simulink model "mcb_pmsm_foc_hall_f28379d"  (R2023b)
settings: Solver=FixedStepDiscrete  StartTime=0.0  StopTime=8  RelTol=1e-3  EnableMultiTasking=on
InitFcn:
  | mcb_pmsm_foc_hall_f28379d_data;
model workspace (MAT data in the model file):
  encoderResolution = 2000
  hallOffset = '0.5'
  indexOffset = 850
  polePairs = '4'
values from neighbouring files (symbols this model uses):
  dataType = 'single'    [mcb_pmsm_foc_hall_f28069m_data.m]    (also in mcb_pmsm_foc_hall_f28379d_data.m)
  inverter = mcb_SetInverterParameters('DRV8312-C2-KIT')    [mcb_pmsm_foc_hall_f28069m_data.m]    (also in mcb_pmsm_foc_hall_f28379d_data.m = mcb_updateInverterParameters(pmsm,inverter,target))
  PI_params = mcb_SetControllerParameters(pmsm,inverter,PU_System,T_pwm,Ts,Ts_speed)    [mcb_pmsm_foc_hall_f28069m_data.m]    (also in mcb_pmsm_foc_hall_f28379d_data.m)
  pmsm = mcb_SetPMSMMotorParameters('BLY171D')    [mcb_pmsm_foc_hall_f28069m_data.m]    (also in mcb_pmsm_foc_hall_f28379d_data.m = mcb_SetPMSMMotorParameters('custom'))
  PU_System = mcb_SetPUSystem(pmsm,inverter)    [mcb_pmsm_foc_hall_f28069m_data.m]    (also in mcb_pmsm_foc_hall_f28379d_data.m)
  target = mcb_SetProcessorDetails('F28069M',PWM_frequency)    [mcb_pmsm_foc_hall_f28069m_data.m]    (also in mcb_pmsm_foc_hall_f28379d_data.m = mcb_SetProcessorDetails('F28379D',PWM_frequency))
  Ts = T_pwm    (= 5e-05)    [mcb_pmsm_foc_hall_f28069m_data.m]    (also in mcb_pmsm_foc_hall_f28379d_data.m)
  Ts_motor = T_pwm/2    (= 2.5e-05)    [mcb_pmsm_foc_hall_f28069m_data.m]    (also in mcb_pmsm_foc_hall_f28379d_data.m)
  Ts_simulink = T_pwm/2    (= 2.5e-05)    [mcb_pmsm_foc_hall_f28069m_data.m]    (also in mcb_pmsm_foc_hall_f28379d_data.m)
  Ts_speed = 10*Ts    (= 0.0005)    [mcb_pmsm_foc_hall_f28069m_data.m]    (also in mcb_pmsm_foc_hall_f28379d_data.m)
undefined symbols (not defined in the file or in its folder): DiscIntNeverNeededParam, Down, GPTRIP1SEL, GPTRIP2SEL, Ts_sensor, TZ1, TZ2, Up
libraries: simulink x37, mcbpositiondecoderlib x12, mcbcontrolslib x11, idelinklib_common x8, c280xlib x8, c2802xlib x7, svdschedulerlib x5, slpidlib x4, c2837xDlib x3, svdutilitieslib x1, mcbplantlib x1, autolibpmsmexterior x1
(part 2 of 4)

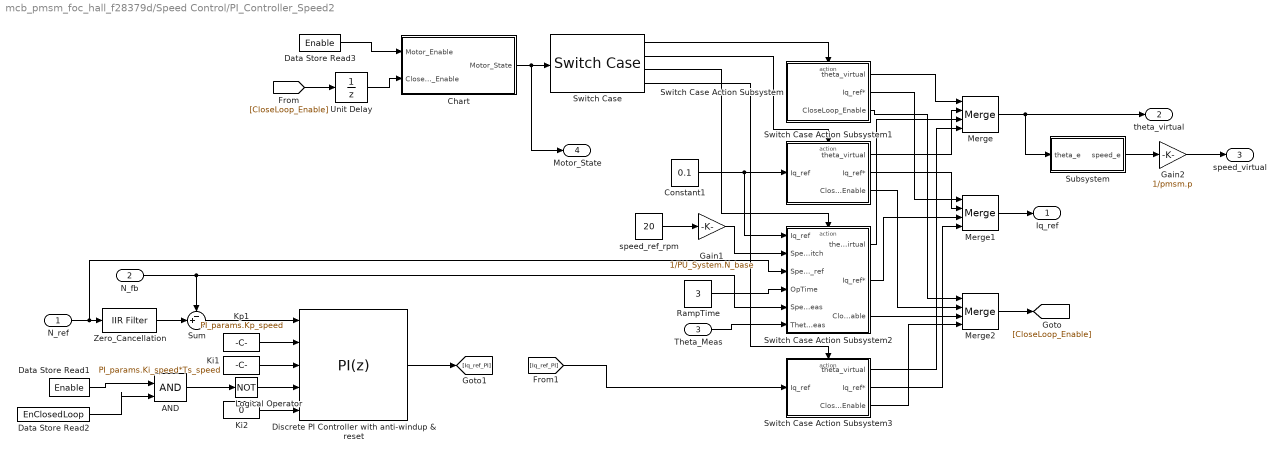
== system mcb_pmsm_foc_hall_f28379d/Speed Control/PI_Controller_Speed2 ==
  N_ref : Inport
  N_fb : Inport  Port=2
  Theta_Meas : Inport  Port=3
  AND : Logic  IconShape=distinctive  AllPortsSameDT=off  OutDataTypeStr=boolean
  Chart : Stateflow chart  TreatAsAtomicUnit=on
  Constant1 : Constant  Value=0.1  OutDataTypeStr=single
  Data Store Read2 : DataStoreRead  DataStoreName=EnClosedLoop  IndexOptions=Index vector (dialog)  Indices=1  OutputSizes=1
  Data Store Read1 : DataStoreRead  DataStoreName=Enable  IndexOptions=Index vector (dialog)  Indices=1  OutputSizes=1
  Data Store Read3 : DataStoreRead  DataStoreName=Enable  IndexOptions=Index vector (dialog)  Indices=1  OutputSizes=1
  Discrete PI Controller with anti-windup & reset : slpidlib/PID Controller  Controller=PI  Form=Parallel  TimeDomain=Discrete-time  UseExternalTs=off  SampleTime=-1  IntegratorMethod=Forward Euler  FilterMethod=Forward Euler  ControllerParametersSource=external  P=1  I=1  UseKiTs=on  D=0  N=100  UseFilter=on  TunerSelectOption=Transfer Function Based (PID Tuner App)  InitialConditionSource=external  InitialConditionForIntegrator=0  InitialConditionForFilter=0  DifferentiatorICPrevScaledInput=0  ExternalReset=level  TrackingMode=off  Kt=1  LimitOutput=on  SatLimitsSource=internal  UpperSaturationLimit=1  LowerSaturationLimit=-1  LinearizeAsGain=on  AntiWindupMode=clamping  Kb=1  LimitIntegrator=off  UpperIntegratorSaturationLimit=inf  LowerIntegratorSaturationLimit=-inf  RndMeth=Simplest  POutMin=[]  POutMax=[]  IOutMin=[]  IOutMax=[]  DOutMin=[]  DOutMax=[]  NOutMin=[]  NOutMax=[]  SumOutMin=[]  SumOutMax=[]  SaturationOutDataTypeStr=Inherit: Inherit via back propagation  SaturationOutMin=[]  SaturationOutMax=[]  PParamMin=[]  PParamMax=[]  IParamMin=[]  IParamMax=[]  DParamMin=[]  DParamMax=[]  NParamMin=[]  NParamMax=[]  KbParamMin=[]  KbParamMax=[]  KtParamMin=[]  KtParamMax=[]  KbOutMin=[]  KbOutMax=[]  KtOutMin=[]  KtOutMax=[]  IntegratorOutMin=[]  IntegratorOutMax=[]  FilterOutMin=[]  FilterOutMax=[]  SumI1OutMin=[]  SumI1OutMax=[]  SumI2OutMin=[]  SumI2OutMax=[]  SumI3OutMin=[]  SumI3OutMax=[]  SumI4OutMin=[]  SumI4OutMax=[]  SumDOutMin=[]  SumDOutMax=[]  DifferentiatorOutMin=[]  DifferentiatorOutMax=[]  FilterDiffOutCoefMin=[]  FilterDiffOutCoefMax=[]  ReciprocalOutMin=[]  ReciprocalOutMax=[]  SumDenOutMin=[]  SumDenOutMax=[]  SumNumOutMin=[]  SumNumOutMax=[]  DivideOutMin=[]  DivideOutMax=[]  UdiffTsProdOutMin=[]  UdiffTsProdOutMax=[]  NTsProdOutMin=[]  NTsProdOutMax=[]  UintegralTsProdOutMin=[]  UintegralTsProdOutMax=[]  UngainTsProdOutMin=[]  UngainTsProdOutMax=[]  ClampingZeroOutDataTypeStr=Inherit: Inherit via back propagation  ClampingZeroOutMin=[]  ClampingZeroOutMax=[]  FilterDenConstantOutDataTypeStr=Inherit: Inherit via back propagation  FilterDenConstantOutMin=[]  FilterDenConstantOutMax=[]  PCopyOutDataTypeStr=Inherit: Inherit via back propagation  PCopyOutMin=[]  PCopyOutMax=[]  NCopyOutDataTypeStr=Inherit: Inherit via back propagation  NCopyOutMin=[]  NCopyOutMax=[]  IntegratorContinuousStateAttributes=''  IntegratorStateMustResolveToSignalObject=off  IntegratorRTWStateStorageClass=Auto  FilterContinuousStateAttributes=''  FilterStateMustResolveToSignalObject=off  FilterRTWStateStorageClass=Auto  ParallelPVariant=ExternalParameters  IdealPVariant=Disabled  IVariant=ExternalParameters  DVariant=Disabled  IntegratorVariant=Discrete  SatVariant=Enabled  AWVariant=DiscClampingParallel  PCopyVariant=Disabled  TRVariant=Disabled  FdbkBlocksVariant=Forward  IdealPFdbkVariant=Disabled  SatFdbkVariant=Disabled  DerivativeFilterVariant=Disabled  NVariant=Disabled  NCopyVariant=Disabled_SignalSpec  FilterICVariant=Disabled  IntegratorICVariant=ExternalICs  ExternalResetVariant=ExternalReset  TRSumVariant=Passthrough  SumFdbkVariant=Disabled  SumVariant=Sum_PI  TsampFilterVariant=InternalTs  TsampNgainVariant=Passthrough  TsampIntegralVariant=Disabled_SignalSpec  ExternalSaturationOutDataTypeStr=Inherit: Same as second input
      settings: LibrarySourceBlock=mcbcontrolslib/PI Controller
  Gain1 : Gain  Gain=1/PU_System.N_base
  Gain2 : Gain  Gain=1/pmsm.p
  Ki1 : Constant  Value=PI_params.Ki_speed*Ts_speed  OutDataTypeStr=dataType  SampleTime=-1
  Ki2 : Constant  Value=0  OutDataTypeStr=dataType  SampleTime=-1
  Kp1 : Constant  Value=PI_params.Kp_speed  OutDataTypeStr=dataType  SampleTime=-1
  Logical Operator : Logic  Operator=NOT  IconShape=distinctive  AllPortsSameDT=off  OutDataTypeStr=boolean
  Merge : Merge  Inputs=4
  Merge1 : Merge  Inputs=4
  Merge2 : Merge  Inputs=4
  RampTime : Constant  Value=3  OutDataTypeStr=single
  Subsystem : Subsystem
  Sum : Sum  Inputs=-+|  OutDataTypeStr=Inherit: Same as first input
  Switch Case : SwitchCase  CaseConditions={1,2,3,4}  ShowDefaultCase=off
  Switch Case Action Subsystem : Subsystem  TreatAsAtomicUnit=on
  Switch Case Action Subsystem1 : Subsystem  TreatAsAtomicUnit=on
  Switch Case Action Subsystem2 : Subsystem  TreatAsAtomicUnit=on
  Switch Case Action Subsystem3 : Subsystem  TreatAsAtomicUnit=on
  Unit Delay : UnitDelay  SampleTime=-1  HasFrameUpgradeWarning=on
  Zero_Cancellation : mcbcontrolslib/IIR Filter  VariantControl=Low Pass Filter  VariantSelect=Low-pass  Filter_constant=0.01*(Ts_speed/Ts)  advancedSettings=off  Ts=50e-6  cutOff_freq=1
  speed_ref_rpm : Constant  Value=20  OutDataTypeStr=double
  Iq_ref : Outport  VectorParamsAs1DForOutWhenUnconnected=off
  theta_virtual : Outport  Port=2  VectorParamsAs1DForOutWhenUnconnected=off
  speed_virtual : Outport  Port=3  VectorParamsAs1DForOutWhenUnconnected=off
  Motor_State : Outport  Port=4
  wires:
  Ki1/1 -> Discrete PI Controller with anti-windup & reset/3
  Kp1/1 -> Discrete PI Controller with anti-windup & reset/2
  N_ref/1 -> Switch Case Action Subsystem2/3(Speed_ref), Zero_Cancellation/1
  Sum/1 -> Discrete PI Controller with anti-windup & reset/1
  Logical Operator/1 -> Discrete PI Controller with anti-windup & reset/4
  Ki2/1 -> Discrete PI Controller with anti-windup & reset/5
  Data Store Read1/1 -> AND/1
  Data Store Read2/1 -> AND/2
  AND/1 -> Logical Operator/1
  Data Store Read3/1 -> Chart/1(Motor_Enable)
  Switch Case/1 -> Switch Case Action Subsystem/Action
  Switch Case/2 -> Switch Case Action Subsystem1/Action
  Switch Case/3 -> Switch Case Action Subsystem2/Action
  Switch Case Action Subsystem/1(theta_virtual) -> Merge/1
  Switch Case Action Subsystem1/1(theta_virtual) -> Merge/2
  Switch Case Action Subsystem2/1(theta_virtual) -> Merge/3
  Switch Case Action Subsystem3/1(theta_virtual) -> Merge/4
  Switch Case Action Subsystem/2(Iq_ref*) -> Merge1/1
  Switch Case Action Subsystem1/2(Iq_ref*) -> Merge1/2
  Switch Case Action Subsystem2/2(Iq_ref*) -> Merge1/3
  Switch Case Action Subsystem3/2(Iq_ref*) -> Merge1/4
  Switch Case/4 -> Switch Case Action Subsystem3/Action
  Gain1/1 -> Switch Case Action Subsystem2/2(Speed_switch)
  RampTime/1 -> Switch Case Action Subsystem2/4(OpTime)
  Merge1/1 -> Iq_ref/1
  Theta_Meas/1 -> Switch Case Action Subsystem2/6(Theta_Meas)
  Zero_Cancellation/1 -> Sum/2
  N_fb/1 -> Sum/1, Switch Case Action Subsystem2/5(Speed_Meas)
  [CloseLoop_Enable] -> Unit Delay/1
  Merge2/1 -> [CloseLoop_Enable]
  Switch Case Action Subsystem/3(CloseLoop_Enable) -> Merge2/1
  Switch Case Action Subsystem1/3(CloseLoop_Enable) -> Merge2/2
  Switch Case Action Subsystem2/3(CloseLoop_Enable) -> Merge2/3
  Switch Case Action Subsystem3/3(CloseLoop_Enable) -> Merge2/4
  Unit Delay/1 -> Chart/2(CloseLoop_Enable)
  speed_ref_rpm/1 -> Gain1/1
  Constant1/1 -> Switch Case Action Subsystem1/1(Iq_ref), Switch Case Action Subsystem2/1(Iq_ref)
  Discrete PI Controller with anti-windup & reset/1 -> [Iq_ref_PI]
  [Iq_ref_PI] -> Switch Case Action Subsystem3/1(Iq_ref)
  Chart/1(Motor_State) -> Motor_State/1, Switch Case/1
  Merge/1 -> theta_virtual/1, Subsystem/1(theta_e)
  Subsystem/1(speed_e) -> Gain2/1
  Gain2/1 -> speed_virtual/1

== system mcb_pmsm_foc_hall_f28379d/Speed Control/Speed_Ref_Selector ==
  Speed_Ref_In : Inport
  Speed_Ref_Open : Inport  Port=2
  Data Store Read1 : DataStoreRead  DataStoreName=Enable  IndexOptions=Index vector (dialog)  Indices=1  OutputSizes=1
  Switch : Switch  Criteria=u2 > Threshold  Threshold=0.5  SaturateOnIntegerOverflow=off  InputSameDT=off
  Speed_Ref_PU : Outport
  wires:
  Switch/1 -> Speed_Ref_PU/1
  Data Store Read1/1 -> Switch/2
  Speed_Ref_Open/1 -> Switch/3
  Speed_Ref_In/1 -> Switch/1

== system mcb_pmsm_foc_hall_f28379d/Current Control/Control_System/Current_Controllers ==
  Id : Inport
  Iq : Inport  Port=2
  Idq_ref_PU : Inport  Port=3
  DQ Limiter : mcbcontrolslib/DQ Limiter  satMethodInputType=Specify via dialog  satMethodSelected=D-Q equivalence  satLimitInputType=Specify via dialog  Vmax=0.95
  Demux : Demux  Outputs=2
  Mux : Mux
  PI_Controller_Id : Subsystem
  PI_Controller_Iq : Subsystem
  Terminator : Terminator
  Vd_ref : Outport  VectorParamsAs1DForOutWhenUnconnected=off
  Vq_ref : Outport  Port=2  VectorParamsAs1DForOutWhenUnconnected=off
  Idq : Outport  Port=3  VectorParamsAs1DForOutWhenUnconnected=off
  wires:
  Iq/1 -> Mux/4, PI_Controller_Iq/2(I_fb)  "Iq_fb"
  PI_Controller_Iq/1(V_ref) -> DQ Limiter/2
  PI_Controller_Id/1(V_ref) -> DQ Limiter/1
  Id/1 -> Mux/2, PI_Controller_Id/2(I_fb)  "Id_fb"
  Idq_ref_PU/1 -> Demux/1
  DQ Limiter/1 -> Vd_ref/1
  DQ Limiter/2 -> Vq_ref/1
  DQ Limiter/3 -> Terminator/1
  Demux/1 -> Mux/1, PI_Controller_Id/1(I_ref)  "Id_Ref"
  Demux/2 -> Mux/3, PI_Controller_Iq/1(I_ref)  "Iq_Ref"
  Mux/1 -> Idq/1

== system mcb_pmsm_foc_hall_f28379d/Current Control/Error Trigger/堵转 ==
  In1 : Inport
  Action Port : ActionPort  ActionPortLabel=if((u1 > 0) & (u2 > u3) & (u4 ~= 0))
  Constant1 : Constant  Value=0.1
  Discrete Pulse Generator : DiscretePulseGenerator  Amplitude=0.2  Period=38  PulseWidth=19  SampleTime=-1
  Subtract : Sum  Inputs=+-
  ERROR : Outport
  Vd : Outport  Port=2
  wires:
  In1/1 -> ERROR/1
  Subtract/1 -> Vd/1
  Discrete Pulse Generator/1 -> Subtract/1
  Constant1/1 -> Subtract/2

== system mcb_pmsm_foc_hall_f28379d/Current Control/Error Trigger/正常运行 ==
  In1 : Inport
  Action Port : ActionPort  ActionPortLabel=else
  Constant : Constant  Value=0
  ERROR : Outport
  Vd : Outport  Port=2
  wires:
  In1/1 -> ERROR/1
  Constant/1 -> Vd/1

== system mcb_pmsm_foc_hall_f28379d/Current Control/Input Scaling/Read_Sensor (codegen) ==
  Iab_meas_ADC : Inport
  Iab_Sim : Inport  Port=2
  Pos_Sim : Inport  Port=3
  Calculate Position from Hall : Subsystem
  Convert ADC value to PU : Subsystem
  Terminator : Terminator
  Terminator1 : Terminator
  Iab_meas_PU : Outport  VectorParamsAs1DForOutWhenUnconnected=off
  Pos_PU : Outport  Port=2  InitialOutput=0  VectorParamsAs1DForOutWhenUnconnected=off
  speed_PU : Outport  Port=3  InitialOutput=0  VectorParamsAs1DForOutWhenUnconnected=off
  ADC : Outport  Port=4  VectorParamsAs1DForOutWhenUnconnected=off
  wires:
  Iab_Sim/1 -> Terminator/1
  Pos_Sim/1 -> Terminator1/1
  Iab_meas_ADC/1 -> Convert ADC value to PU/1(Iab_meas_ADC)
  Convert ADC value to PU/1(Iab_meas_PU) -> Iab_meas_PU/1
  Calculate Position from Hall/1(Pos_PU) -> Pos_PU/1
  Calculate Position from Hall/2(Speed_PU) -> speed_PU/1
  Convert ADC value to PU/2(Iab_meas_PU1) -> ADC/1

== system mcb_pmsm_foc_hall_f28379d/Current Control/Input Scaling/Read_Sensor (sim) ==
  Iab_meas_ADC : Inport  OutDataTypeStr=uint16
  Iab_Sim : Inport  Port=2
  Pos_Sim : Inport  Port=3
  Convert ADC value to PU : Subsystem
  Convert meas angle to PU : Subsystem
  Terminator : Terminator
  Iab_meas_PU : Outport  VectorParamsAs1DForOutWhenUnconnected=off
  Pos_PU : Outport  Port=2  InitialOutput=0  VectorParamsAs1DForOutWhenUnconnected=off
  speed_PU : Outport  Port=3  InitialOutput=0  VectorParamsAs1DForOutWhenUnconnected=off
  ADC : Outport  Port=4  VectorParamsAs1DForOutWhenUnconnected=off
  wires:
  Iab_meas_ADC/1 -> Terminator/1
  Iab_Sim/1 -> Convert ADC value to PU/1(Iab_meas_ADC)
  Convert ADC value to PU/1(Iab_meas_PU) -> Iab_meas_PU/1
  Pos_Sim/1 -> Convert meas angle to PU/1(Pos_Sim)  "Iab_fb"
  Convert meas angle to PU/1(Theta) -> Pos_PU/1
  Convert meas angle to PU/2(Speed) -> speed_PU/1

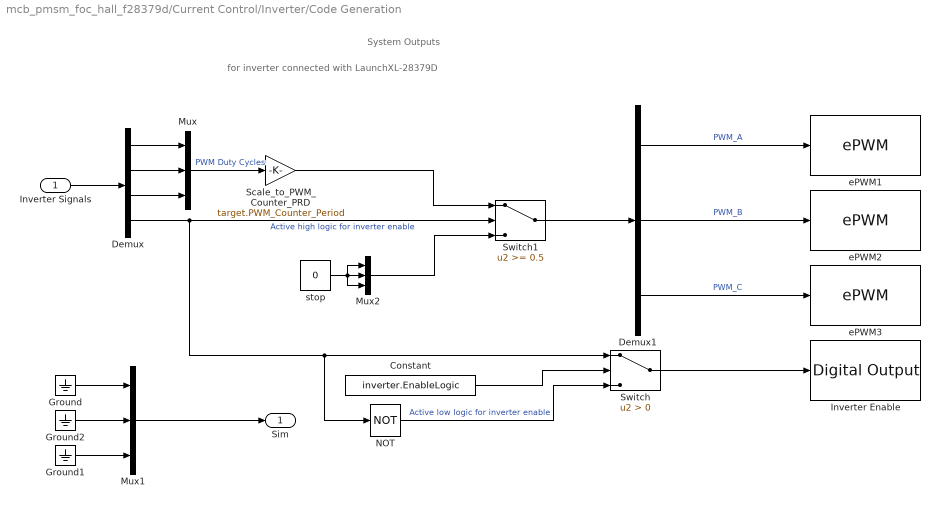
== system mcb_pmsm_foc_hall_f28379d/Current Control/Inverter/Code Generation ==
  note: for inverter connected with LaunchXL-28379D
  note: System Outputs
  Inverter Signals : Inport
  Constant : Constant  Value=inverter.EnableLogic
  Demux : Demux
  Demux1 : Demux  Outputs=3
  Ground : Ground
  Ground1 : Ground
  Ground2 : Ground
  Inverter Enable : c2837xDlib/Digital Output  GPIO_Number=GPIO120~GPIO127  GPIO_Bit0=off  GPIO_BIT0_Toggle=off  GPIO_Bit1=off  GPIO_BIT1_Toggle=off  GPIO_Bit2=off  GPIO_BIT2_Toggle=off  GPIO_Bit3=off  GPIO_BIT3_Toggle=off  GPIO_Bit4=on  GPIO_BIT4_Toggle=off  GPIO_Bit5=off  GPIO_BIT5_Toggle=off  GPIO_Bit6=off  GPIO_BIT6_Toggle=off  GPIO_Bit7=off  GPIO_BIT7_Toggle=off
  Mux : Mux  Inputs=3
  Mux1 : Mux  Inputs=3
  Mux2 : Mux  Inputs=3
  NOT : Logic  Operator=NOT  IconShape=distinctive  AllPortsSameDT=off  OutDataTypeStr=boolean
  Scale_to_PWM_Counter_PRD : Gain  Gain=target.PWM_Counter_Period  OutDataTypeStr=uint16  RndMeth=Simplest
  Switch : Switch  Criteria=u2 > Threshold  SaturateOnIntegerOverflow=off  InputSameDT=off
  Switch1 : Switch  Threshold=0.5  SaturateOnIntegerOverflow=off  InputSameDT=off
  ePWM1 : c2802xlib/ePWM  PwmType=C2000_Type4  useModule=ePWM1  ePWMxLINKTBPRD=Not Linked  periodUnits=Clock cycles  timerSource=Specify via dialog  timerPeriod_clk=target.PWM_Counter_Period  timerPeriod_sec=0.0001  tbshadow=Counter equals to zero  countingMode=Up-Down  phaseActiveEnable=Disable  phaseDirection=Count down after sync  phaseActive=0  synchronizationEnable=off  dcaevt1Sync=off  dcbevt1Sync=off  synchronizationOption=Counter equals to zero (CTR=Zero)  dcbevt1SyncOut=off  dcaevt1SyncOut=off  cmpdSyncOut=off  cmpcSyncOut=off  cmpbSyncOut=off  zeroSyncOut=on  swfSyncOut=off  perSynchronizationOption=Counter equals to period (CTR=PRD)  clockPrescale=1  HSclockPrescale=1  enswap=off  ePWMxAStatus=on  ePWMxAactionLogic1=Do nothing  ePWMxAactionLogic2=Do nothing  ePWMxAactionLogic3=Clear  ePWMxAactionLogic4=Set  ePWMxAactionLogic5=Do nothing  ePWMxAactionLogic6=Do nothing  ePWMxACSFenable=off  ePWMxACSFvalue=Forcing disable  ePWMxASFreload=Zero  ePWMxBStatus=off  ePWMxBactionLogic1=Set  ePWMxBactionLogic2=Clear  ePWMxBactionLogic3=Do nothing  ePWMxBactionLogic4=Do nothing  ePWMxBactionLogic5=Clear  ePWMxBactionLogic6=Set  ePWMxBCSFenable=off  ePWMxBCSFvalue=Forcing disable  ePWMxBSFreload=Zero  ePWNxBOutWay=off  ePWMxLINKCMPA=Not Linked  CMPAUnits=Clock cycles  CMPASource=Input port  CMPAValue_per=50  CMPAValue_clk=floor(target.PWM_Counter_Period/2+1)  enCMPAshadow=Counter equals to zero (CTR=Zero)  ePWMxLINKCMPB=Not Linked  CMPBUnits=Clock cycles  CMPBSource=Specify via dialog  CMPBValue_per=50  CMPBValue_clk=floor(target.PWM_Counter_Period/2+1)  enCMPBshadow=Counter equals to zero (CTR=Zero)  ePWMxLINKCMPC=Not Linked  CMPCUnits=Clock cycles  CMPCSource=Specify via dialog  CMPCValue_per=50  CMPCValue_clk=32000  enCMPCshadow=Counter equals to zero (CTR=Zero)  ePWMxLINKCMPD=Not Linked  CMPDUnits=Clock cycles  CMPDSource=Specify via dialog  CMPDValue_per=50  CMPDValue_clk=32000  enCMPDshadow=Counter equals to zero (CTR=Zero)  enableDBePWMxA=on  enableDBePWMxB=on  enhalfcycle=off  DBpolarity=Active high complementary (AHC)  DBedgeDelay=Positive  DBSource_ePWMxA=ePWMxA  DBSource_ePWMxB=ePWMxA  DBPeriodUnits=Clock cycles  DBperiodSource=Specify via dialog  REDperiod=15  FEDperiod=15  REDperiod_sec=0  FEDperiod_sec=0  LoadModeDBRED=Immediate without using shadow  LoadModeDBFED=Immediate without using shadow  adcstartModuleA=on  adcrequestEventA=First event  adcstartEventA=Digital Compare Module A Event 1 start of conversion (DCAEVT1.soc)  adcstartEventA_type2=Counter equals to period (CTR=PRD)  adcstartModuleB=off  adcrequestEventB=First event  adcstartEventB=Counter equals to zero (CTR=Zero)  adcstartEventB_type2=Counter equals to zero (CTR=Zero)  intEn=off  intPrd=First event  intSel=Counter equals to zero (CTR=Zero)  intSel_type2=Counter equals to zero (CTR=Zero)  hrpe=off  enHRPWM=off  HRPWM_LoadMode=Counter equals to period (CTR=PRD)  HRPWM_CTLMode=Duty or Period control mode  HRPWM_EDGMode=Both edge  hrpeb=off  enHRPWMB=off  HRPWM_LoadModeB=Counter equals to zero (CTR=ZERO)  HRPWM_CTLModeB=Duty or Period control mode  HRPWM_EDGModeB=Both edge  enHRDBRED=off  enHRDBFED=off  enSFO=on  enautoconv=on  chopperEnable=off  chopperFrequency=1  chopperFirstwidth=1  chopperDuty=12.5%  tripZonesource=Specify via dialog  tzselOSHT1=off  tzselOSHT2=off  tzselOSHT3=off  tzselOSHDCAEV1=off  tzselOSHDCBEV1=off  tzselCBC1=off  tzselCBC2=off  tzselCBC3=off  tzselCBCDCAEV2=off  tzselCBCDCBEV2=off  tzselOSHT4=off  tzselOSHT5=off  tzselOSHT6=off  tzselCBC4=off  tzselCBC5=off  tzselCBC6=off  enTzOstIntr=off  enTzCbcIntr=off  enTzDCAEVT1Intr=off  enTzDCAEVT2Intr=off  enTzDCBEVT1Intr=off  enTzDCBEVT2Intr=off  ePWMxAforced=No action  ePWMxBforced=No action  DCAEVT1forced=No action  DCBEVT1forced=No action  DCAEVT2forced=No action  DCBEVT2forced=No action  dcah=Trip Zone 1 input (TZ1)  dcal=Trip Zone 2 input (TZ2)  dcbh=Trip Zone 1 input (TZ1)  dcbl=Trip Zone 2 input (TZ2)  dcah_type2=GPTRIP1SEL/(TZ1)  dcal_type2=GPTRIP2SEL/(TZ2)  dcbh_type2=GPTRIP1SEL/(TZ1)  dcbl_type2=GPTRIP2SEL/(TZ2)  gendcaevt1=Event disabled  gendcaevt2=Event disabled  gendcbevt1=Event disabled  gendcbevt2=Event disabled  dcaevt1src=DCAEVT1 with sync  dcaevt2src=DCAEVT2 with sync  dcbevt1src=DCBEVT1 with sync  dcbevt2src=DCBEVT2 with sync  pulsesel=Counter equals to zero (CTR=Zero)  blankinv=off  blankoffset=0  blankwidth=0  evsrcsel=Filtered version of DCAEVT1 (DCAEVT1FILT)  encape=off
  ePWM2 : c2802xlib/ePWM  PwmType=C2000_Type4  useModule=ePWM2  ePWMxLINKTBPRD=Not Linked  periodUnits=Clock cycles  timerSource=Specify via dialog  timerPeriod_clk=target.PWM_Counter_Period  timerPeriod_sec=0.0001  tbshadow=Counter equals to zero  countingMode=Up-Down  phaseActiveEnable=Set counter to phase value specified via dialog  phaseDirection=Count up after sync  phaseActive=0  synchronizationEnable=off  dcaevt1Sync=off  dcbevt1Sync=off  synchronizationOption=Pass through (EPWMxSYNCI or SWFSYNC)  dcbevt1SyncOut=off  dcaevt1SyncOut=off  cmpdSyncOut=off  cmpcSyncOut=off  cmpbSyncOut=off  zeroSyncOut=off  swfSyncOut=on  perSynchronizationOption=Counter equals to period (CTR=PRD)  clockPrescale=1  HSclockPrescale=1  enswap=off  ePWMxAStatus=on  ePWMxAactionLogic1=Do nothing  ePWMxAactionLogic2=Do nothing  ePWMxAactionLogic3=Clear  ePWMxAactionLogic4=Set  ePWMxAactionLogic5=Do nothing  ePWMxAactionLogic6=Do nothing  ePWMxACSFenable=off  ePWMxACSFvalue=Forcing disable  ePWMxASFreload=Zero  ePWMxBStatus=off  ePWMxBactionLogic1=Set  ePWMxBactionLogic2=Clear  ePWMxBactionLogic3=Do nothing  ePWMxBactionLogic4=Do nothing  ePWMxBactionLogic5=Clear  ePWMxBactionLogic6=Set  ePWMxBCSFenable=off  ePWMxBCSFvalue=Forcing disable  ePWMxBSFreload=Zero  ePWNxBOutWay=off  ePWMxLINKCMPA=Not Linked  CMPAUnits=Clock cycles  CMPASource=Input port  CMPAValue_per=50  CMPAValue_clk=floor(target.PWM_Counter_Period/2+1)  enCMPAshadow=Counter equals to zero (CTR=Zero)  ePWMxLINKCMPB=Not Linked  CMPBUnits=Clock cycles  CMPBSource=Specify via dialog  CMPBValue_per=50  CMPBValue_clk=floor(target.PWM_Counter_Period/2+1)  enCMPBshadow=Counter equals to zero (CTR=Zero)  ePWMxLINKCMPC=Not Linked  CMPCUnits=Clock cycles  CMPCSource=Specify via dialog  CMPCValue_per=50  CMPCValue_clk=32000  enCMPCshadow=Counter equals to zero (CTR=Zero)  ePWMxLINKCMPD=Not Linked  CMPDUnits=Clock cycles  CMPDSource=Specify via dialog  CMPDValue_per=50  CMPDValue_clk=32000  enCMPDshadow=Counter equals to zero (CTR=Zero)  enableDBePWMxA=on  enableDBePWMxB=on  enhalfcycle=off  DBpolarity=Active high complementary (AHC)  DBedgeDelay=Positive  DBSource_ePWMxA=ePWMxA  DBSource_ePWMxB=ePWMxA  DBPeriodUnits=Clock cycles  DBperiodSource=Specify via dialog  REDperiod=15  FEDperiod=15  REDperiod_sec=0  FEDperiod_sec=0  LoadModeDBRED=Immediate without using shadow  LoadModeDBFED=Immediate without using shadow  adcstartModuleA=off  adcrequestEventA=First event  adcstartEventA=Digital Compare Module A Event 1 start of conversion (DCAEVT1.soc)  adcstartEventA_type2=Counter equals to period (CTR=PRD)  adcstartModuleB=off  adcrequestEventB=First event  adcstartEventB=Counter equals to zero (CTR=Zero)  adcstartEventB_type2=Counter equals to zero (CTR=Zero)  intEn=off  intPrd=First event  intSel=Counter equals to zero (CTR=Zero)  intSel_type2=Counter equals to zero (CTR=Zero)  hrpe=off  enHRPWM=off  HRPWM_LoadMode=Counter equals to period (CTR=PRD)  HRPWM_CTLMode=Duty or Period control mode  HRPWM_EDGMode=Both edge  hrpeb=off  enHRPWMB=off  HRPWM_LoadModeB=Counter equals to zero (CTR=ZERO)  HRPWM_CTLModeB=Duty or Period control mode  HRPWM_EDGModeB=Both edge  enHRDBRED=off  enHRDBFED=off  enSFO=on  enautoconv=on  chopperEnable=off  chopperFrequency=1  chopperFirstwidth=1  chopperDuty=12.5%  tripZonesource=Specify via dialog  tzselOSHT1=off  tzselOSHT2=off  tzselOSHT3=off  tzselOSHDCAEV1=off  tzselOSHDCBEV1=off  tzselCBC1=off  tzselCBC2=off  tzselCBC3=off  tzselCBCDCAEV2=off  tzselCBCDCBEV2=off  tzselOSHT4=off  tzselOSHT5=off  tzselOSHT6=off  tzselCBC4=off  tzselCBC5=off  tzselCBC6=off  enTzOstIntr=off  enTzCbcIntr=off  enTzDCAEVT1Intr=off  enTzDCAEVT2Intr=off  enTzDCBEVT1Intr=off  enTzDCBEVT2Intr=off  ePWMxAforced=No action  ePWMxBforced=No action  DCAEVT1forced=No action  DCBEVT1forced=No action  DCAEVT2forced=No action  DCBEVT2forced=No action  dcah=Trip Zone 1 input (TZ1)  dcal=Trip Zone 2 input (TZ2)  dcbh=Trip Zone 1 input (TZ1)  dcbl=Trip Zone 2 input (TZ2)  dcah_type2=GPTRIP1SEL/(TZ1)  dcal_type2=GPTRIP2SEL/(TZ2)  dcbh_type2=GPTRIP1SEL/(TZ1)  dcbl_type2=GPTRIP2SEL/(TZ2)  gendcaevt1=Event disabled  gendcaevt2=Event disabled  gendcbevt1=Event disabled  gendcbevt2=Event disabled  dcaevt1src=DCAEVT1 with sync  dcaevt2src=DCAEVT2 with sync  dcbevt1src=DCBEVT1 with sync  dcbevt2src=DCBEVT2 with sync  pulsesel=Counter equals to zero (CTR=Zero)  blankinv=off  blankoffset=0  blankwidth=0  evsrcsel=Filtered version of DCAEVT1 (DCAEVT1FILT)  encape=off
  ePWM3 : c2802xlib/ePWM  PwmType=C2000_Type4  useModule=ePWM3  ePWMxLINKTBPRD=Not Linked  periodUnits=Clock cycles  timerSource=Specify via dialog  timerPeriod_clk=target.PWM_Counter_Period  timerPeriod_sec=0.0001  tbshadow=Counter equals to zero  countingMode=Up-Down  phaseActiveEnable=Set counter to phase value specified via dialog  phaseDirection=Count up after sync  phaseActive=0  synchronizationEnable=off  dcaevt1Sync=off  dcbevt1Sync=off  synchronizationOption=Pass through (EPWMxSYNCI or SWFSYNC)  dcbevt1SyncOut=off  dcaevt1SyncOut=off  cmpdSyncOut=off  cmpcSyncOut=off  cmpbSyncOut=off  zeroSyncOut=off  swfSyncOut=on  perSynchronizationOption=Counter equals to period (CTR=PRD)  clockPrescale=1  HSclockPrescale=1  enswap=off  ePWMxAStatus=on  ePWMxAactionLogic1=Do nothing  ePWMxAactionLogic2=Do nothing  ePWMxAactionLogic3=Clear  ePWMxAactionLogic4=Set  ePWMxAactionLogic5=Do nothing  ePWMxAactionLogic6=Do nothing  ePWMxACSFenable=off  ePWMxACSFvalue=Forcing disable  ePWMxASFreload=Zero  ePWMxBStatus=off  ePWMxBactionLogic1=Set  ePWMxBactionLogic2=Clear  ePWMxBactionLogic3=Do nothing  ePWMxBactionLogic4=Do nothing  ePWMxBactionLogic5=Clear  ePWMxBactionLogic6=Set  ePWMxBCSFenable=off  ePWMxBCSFvalue=Forcing disable  ePWMxBSFreload=Zero  ePWNxBOutWay=off  ePWMxLINKCMPA=Not Linked  CMPAUnits=Clock cycles  CMPASource=Input port  CMPAValue_per=50  CMPAValue_clk=floor(target.PWM_Counter_Period/2+1)  enCMPAshadow=Counter equals to zero (CTR=Zero)  ePWMxLINKCMPB=Not Linked  CMPBUnits=Clock cycles  CMPBSource=Specify via dialog  CMPBValue_per=50  CMPBValue_clk=floor(target.PWM_Counter_Period/2+1)  enCMPBshadow=Counter equals to zero (CTR=Zero)  ePWMxLINKCMPC=Not Linked  CMPCUnits=Clock cycles  CMPCSource=Specify via dialog  CMPCValue_per=50  CMPCValue_clk=32000  enCMPCshadow=Counter equals to zero (CTR=Zero)  ePWMxLINKCMPD=Not Linked  CMPDUnits=Clock cycles  CMPDSource=Specify via dialog  CMPDValue_per=50  CMPDValue_clk=32000  enCMPDshadow=Counter equals to zero (CTR=Zero)  enableDBePWMxA=on  enableDBePWMxB=on  enhalfcycle=off  DBpolarity=Active high complementary (AHC)  DBedgeDelay=Positive  DBSource_ePWMxA=ePWMxA  DBSource_ePWMxB=ePWMxA  DBPeriodUnits=Clock cycles  DBperiodSource=Specify via dialog  REDperiod=15  FEDperiod=15  REDperiod_sec=0  FEDperiod_sec=0  LoadModeDBRED=Immediate without using shadow  LoadModeDBFED=Immediate without using shadow  adcstartModuleA=off  adcrequestEventA=First event  adcstartEventA=Digital Compare Module A Event 1 start of conversion (DCAEVT1.soc)  adcstartEventA_type2=Counter equals to period (CTR=PRD)  adcstartModuleB=off  adcrequestEventB=First event  adcstartEventB=Counter equals to zero (CTR=Zero)  adcstartEventB_type2=Counter equals to zero (CTR=Zero)  intEn=off  intPrd=First event  intSel=Counter equals to zero (CTR=Zero)  intSel_type2=Counter equals to zero (CTR=Zero)  hrpe=off  enHRPWM=off  HRPWM_LoadMode=Counter equals to period (CTR=PRD)  HRPWM_CTLMode=Duty or Period control mode  HRPWM_EDGMode=Both edge  hrpeb=off  enHRPWMB=off  HRPWM_LoadModeB=Counter equals to zero (CTR=ZERO)  HRPWM_CTLModeB=Duty or Period control mode  HRPWM_EDGModeB=Both edge  enHRDBRED=off  enHRDBFED=off  enSFO=on  enautoconv=on  chopperEnable=off  chopperFrequency=1  chopperFirstwidth=1  chopperDuty=12.5%  tripZonesource=Specify via dialog  tzselOSHT1=off  tzselOSHT2=off  tzselOSHT3=off  tzselOSHDCAEV1=off  tzselOSHDCBEV1=off  tzselCBC1=off  tzselCBC2=off  tzselCBC3=off  tzselCBCDCAEV2=off  tzselCBCDCBEV2=off  tzselOSHT4=off  tzselOSHT5=off  tzselOSHT6=off  tzselCBC4=off  tzselCBC5=off  tzselCBC6=off  enTzOstIntr=off  enTzCbcIntr=off  enTzDCAEVT1Intr=off  enTzDCAEVT2Intr=off  enTzDCBEVT1Intr=off  enTzDCBEVT2Intr=off  ePWMxAforced=No action  ePWMxBforced=No action  DCAEVT1forced=No action  DCBEVT1forced=No action  DCAEVT2forced=No action  DCBEVT2forced=No action  dcah=Trip Zone 1 input (TZ1)  dcal=Trip Zone 2 input (TZ2)  dcbh=Trip Zone 1 input (TZ1)  dcbl=Trip Zone 2 input (TZ2)  dcah_type2=GPTRIP1SEL/(TZ1)  dcal_type2=GPTRIP2SEL/(TZ2)  dcbh_type2=GPTRIP1SEL/(TZ1)  dcbl_type2=GPTRIP2SEL/(TZ2)  gendcaevt1=Event disabled  gendcaevt2=Event disabled  gendcbevt1=Event disabled  gendcbevt2=Event disabled  dcaevt1src=DCAEVT1 with sync  dcaevt2src=DCAEVT2 with sync  dcbevt1src=DCBEVT1 with sync  dcbevt2src=DCBEVT2 with sync  pulsesel=Counter equals to zero (CTR=Zero)  blankinv=off  blankoffset=0  blankwidth=0  evsrcsel=Filtered version of DCAEVT1 (DCAEVT1FILT)  encape=off
  stop : Constant  Value=0  OutDataTypeStr=uint16
  Sim : Outport  VectorParamsAs1DForOutWhenUnconnected=off
  wires:
  Demux1/3 -> ePWM3/1  "PWM_C"
  Scale_to_PWM_Counter_PRD/1 -> Switch1/1
  Mux2/1 -> Switch1/3
  stop/1 -> Mux2/3, Mux2/2, Mux2/1
  Demux/4 -> Switch1/2, Switch/1, NOT/1  "Active high logic for inverter enable"
  Inverter Signals/1 -> Demux/1
  Demux1/2 -> ePWM2/1  "PWM_B"
  Switch1/1 -> Demux1/1
  Demux1/1 -> ePWM1/1  "PWM_A"
  Mux/1 -> Scale_to_PWM_Counter_PRD/1  "PWM Duty Cycles"
  Ground/1 -> Mux1/1
  Ground1/1 -> Mux1/3
  Ground2/1 -> Mux1/2
  Mux1/1 -> Sim/1
  Demux/1 -> Mux/1
  Demux/2 -> Mux/2
  Demux/3 -> Mux/3
  NOT/1 -> Switch/3  "Active low logic for inverter enable"
  Switch/1 -> Inverter Enable/1
  Constant/1 -> Switch/2

== system mcb_pmsm_foc_hall_f28379d/Current Control/Inverter/Simulation ==
  Inverter Signals : Inport
  Data Type Duplicate : DataTypeDuplicate
  Demux : Demux
  Mux : Mux  Inputs=3
  Mux2 : Mux  Inputs=3
  Switch1 : Switch  Threshold=0.5  RndMeth=Simplest  SaturateOnIntegerOverflow=off  InputSameDT=off
  stop : Constant  Value=0  OutDataTypeStr=Inherit: Inherit via back propagation
  Sim : Outport  VectorParamsAs1DForOutWhenUnconnected=off
  wires:
  stop/1 -> Data Type Duplicate/2, Mux2/1, Mux2/3, Mux2/2
  Mux2/1 -> Switch1/3
  Switch1/1 -> Sim/1
  Inverter Signals/1 -> Demux/1
  Demux/4 -> Switch1/2  "PWM Enable"
  Mux/1 -> Data Type Duplicate/1, Switch1/1  "PWM Duty Cycles"
  Demux/1 -> Mux/1
  Demux/2 -> Mux/2
  Demux/3 -> Mux/3

== system mcb_pmsm_foc_hall_f28379d/Current Control/SCI_Tx/Code Generation ==
  In1 : Inport
  Data_Conditioning_Tx : Subsystem  Variant=on
  Data_Logging : Subsystem
  Demux2 : Demux  Outputs=2
  While Iterator Subsystem : Subsystem  TreatAsAtomicUnit=on
  wires:
  Demux2/2 -> While Iterator Subsystem/2(Iteration)  "SCI_Tx_Iteration"
  Demux2/1 -> While Iterator Subsystem/1(Data)  "SCI_Tx_Data"
  In1/1 -> Data_Conditioning_Tx/1(In1)
  Data_Logging/1(SCI_Tx) -> Demux2/1
  Data_Conditioning_Tx/1(Data_Log) -> Data_Logging/1(Data_Log)

== system mcb_pmsm_foc_hall_f28379d/Current Control/SCI_Tx/Simulation ==
  In1 : Inport
  Demux : Demux  Outputs=2
  Terminator1 : Terminator
  Terminator2 : Terminator
  wires:
  In1/1 -> Demux/1
  Demux/1 -> Terminator1/1
  Demux/2 -> Terminator2/1

== system mcb_pmsm_foc_hall_f28379d/Current Control/Sensor Driver Blocks/Sensor Driver Blocks (codegen) ==
  ADC_B_IN2 : c2802xlib/ADC  blkParamProc=C2000_Type4  ADCModule=B  samplingMode=Single sample mode  ADCResolution=12-bit (Single-ended input)  useSOC1=SOC0  useSOC2=SOC0_SOC1  SOCAcquisitionWindow=15  SOCTriggerSource=ePWM1_ADCSOCA  SOCInterruptTrigger=No ADCINT  Ts=-1  dType=uint16  postInterrupt=on  interruptSel=ADCINT1  ADCINTContinuous=on  endma=off  chdma=1  conv1=ADCINA0  conv2=ADCINA0 and ADCINB0  conv1_Type4=ADCIN2  conv2_Type4=ADCIN0 and ADCIN1
  ADC_C_IN2 : c2802xlib/ADC  blkParamProc=C2000_Type4  ADCModule=C  samplingMode=Single sample mode  ADCResolution=12-bit (Single-ended input)  useSOC1=SOC0  useSOC2=SOC0_SOC1  SOCAcquisitionWindow=15  SOCTriggerSource=ePWM1_ADCSOCA  SOCInterruptTrigger=No ADCINT  Ts=-1  dType=uint16  postInterrupt=off  interruptSel=ADCINT1  ADCINTContinuous=on  endma=off  chdma=1  conv1=ADCINA0  conv2=ADCINA0 and ADCINB0  conv1_Type4=ADCIN2  conv2_Type4=ADCIN0 and ADCIN1
  Mux1 : Mux  Inputs=2
  Iab_Meas_ADC : Outport
  wires:
  ADC_C_IN2/1 -> Mux1/1
  Mux1/1 -> Iab_Meas_ADC/1
  ADC_B_IN2/1 -> Mux1/2

== system mcb_pmsm_foc_hall_f28379d/Current Control/Sensor Driver Blocks/Sensor Driver Blocks (sim) ==
  Ground : Ground
  Iab_Meas_ADC : Outport
  wires:
  Ground/1 -> Iab_Meas_ADC/1

== system mcb_pmsm_foc_hall_f28379d/Current Control/Subsystem/If Action Subsystem ==
  Pos_virtual : Inport
  Vel_virtual : Inport  Port=2
  Action Port : ActionPort  ActionPortLabel=case [ 1 ]:
  Mechanical to Electrical Position : mcbpositiondecoderlib/Mechanical to Electrical Position  PolePairsInputType=Specify via dialog  NrPP=1  selectedRange=Per unit  MechOfstInputType=Specify via dialog  mechOffsetIn=pmsm.PositionOffset  maxAngleIn=1  InputDataType=dataType  VariantSelect=floating-point
  Pos_PU : Outport
  Speed_PU : Outport  Port=2
  wires:
  Mechanical to Electrical Position/1 -> Pos_PU/1
  Pos_virtual/1 -> Mechanical to Electrical Position/1
  Vel_virtual/1 -> Speed_PU/1

== system mcb_pmsm_foc_hall_f28379d/Current Control/Subsystem/If Action Subsystem1 ==
  Pos_Meas : Inport
  speed_Meas : Inport  Port=2
  Action Port : ActionPort  ActionPortLabel=case [ 4 ]:
  Pos_PU : Outport
  Speed_PU : Outport  Port=2
  wires:
  Pos_Meas/1 -> Pos_PU/1
  speed_Meas/1 -> Speed_PU/1

== system mcb_pmsm_foc_hall_f28379d/Current Control/Subsystem/If Action Subsystem2 ==
  Pos_virtual : Inport
  Vel_virtual : Inport  Port=2
  Action Port : ActionPort  ActionPortLabel=case [ 2 ]:
  Mechanical to Electrical Position : mcbpositiondecoderlib/Mechanical to Electrical Position  PolePairsInputType=Specify via dialog  NrPP=1  selectedRange=Per unit  MechOfstInputType=Specify via dialog  mechOffsetIn=pmsm.PositionOffset  maxAngleIn=1  InputDataType=dataType  VariantSelect=floating-point
  Pos_PU : Outport
  Speed_PU : Outport  Port=2
  wires:
  Mechanical to Electrical Position/1 -> Pos_PU/1
  Pos_virtual/1 -> Mechanical to Electrical Position/1
  Vel_virtual/1 -> Speed_PU/1

== system mcb_pmsm_foc_hall_f28379d/Current Control/Subsystem/If Action Subsystem3 ==
  Pos_virtual : Inport
  Vel_virtual : Inport  Port=2
  Action Port : ActionPort  ActionPortLabel=case [ 3 ]:
  Mechanical to Electrical Position : mcbpositiondecoderlib/Mechanical to Electrical Position  PolePairsInputType=Specify via dialog  NrPP=1  selectedRange=Per unit  MechOfstInputType=Specify via dialog  mechOffsetIn=pmsm.PositionOffset  maxAngleIn=1  InputDataType=dataType  VariantSelect=floating-point
  Pos_PU : Outport
  Speed_PU : Outport  Port=2
  wires:
  Mechanical to Electrical Position/1 -> Pos_PU/1
  Pos_virtual/1 -> Mechanical to Electrical Position/1
  Vel_virtual/1 -> Speed_PU/1

== system mcb_pmsm_foc_hall_f28379d/Hall Sensor A/Capture Event Selection/Output 0 ==
  Action Port : ActionPort  ActionPortLabel=else
  Constant : Constant  Value=0  OutDataTypeStr=boolean
  Out1 : Outport
  wires:
  Constant/1 -> Out1/1

== system mcb_pmsm_foc_hall_f28379d/Hall Sensor A/Capture Event Selection/Output 1 ==
  Action Port : ActionPort  ActionPortLabel=if((u1 == 5 | u1 == 3))
  Constant : Constant  OutDataTypeStr=boolean
  Out1 : Outport
  wires:
  Constant/1 -> Out1/1

== system mcb_pmsm_foc_hall_f28379d/Hall Sensor A/HallValidity/CodeGen ==
  Data Type Conversion : DataTypeConversion  OutDataTypeStr=uint32  ConvertRealWorld=Stored Integer (SI)  SaturateOnIntegerOverflow=off  RndMeth=Floor
  Read Halls : Subsystem  mask(Hall sensor reader){sample_time=-1}
      mask prompts: sample_time "Sample time:"
      mask help:
      | This block outputs the state of the 3 hall sensors placed on GPIO54, 55 and 57 of LaunchXL-F28379D board.
      |
      | 0 --> GPIO57 = 0, GPIO55 = 0, GPIO54 = 0
      | 1 --> GPIO57 = 0, GPIO55 = 0, GPIO54 = 1
      | 2 --> GPIO57 = 0, GPIO55 = 1, GPIO54 = 0
      | 3 --> GPIO57 = 0, GPIO55 = 1, GPIO54 = 1
      | 4 --> GPIO57 = 1, GPIO55 = 0, GPIO54 = 0
      | 5 --> GPIO57 = 1, GPIO55 = 0, GPIO54 = 1
      | 6 --> GPIO57 = 1, GPIO55 = 1, GPIO54 = 0
      | 7 --> GPIO57 = 1, GPIO55 = 1, GPIO54 = 1
  Out1 : Outport
  wires:
  Data Type Conversion/1 -> Out1/1
  Read Halls/1(Halls) -> Data Type Conversion/1

== system mcb_pmsm_foc_hall_f28379d/Hall Sensor A/HallValidity/Sim ==
  Data Type Conversion : DataTypeConversion  OutDataTypeStr=uint32  ConvertRealWorld=Stored Integer (SI)  SaturateOnIntegerOverflow=off  RndMeth=Floor
  Ground : Ground
  Out1 : Outport
  wires:
  Data Type Conversion/1 -> Out1/1
  Ground/1 -> Data Type Conversion/1

== system mcb_pmsm_foc_hall_f28379d/Hall Sensor A/eCAP/Code generation ==
  eCAP : c280xlib/eCAP  operatingMode=eCAP  selectCAPx=eCAP1  offsetValue=0  counterSynIn=off  enableCounter=off  syncOutput=Disabled  sampleTime=-1  eventPrescaler=0  selectMode=Continuous  enableOneShot=off  stopValue=Capture Event 2  resetEv1Ts=on  ev1Polarity=Rising Edge  resetEv2Ts=on  ev2Polarity=Falling Edge  resetEv3Ts=off  ev3Polarity=Rising Edge  resetEv4Ts=off  ev4Polarity=Rising Edge  tSCntrDataType=uint32  capEvFlag=off  capFlagDataType=uint16  overFlowFlag=off  overFlowFlagDataType=uint16  periodUnit=Seconds  periodSource=Specify via dialog  waveformPeriod=0.001  dutyUnit=Percentages  dutySource=Specify via dialog  dutyCycle=50  outputPolarity=Active High  enableCEVT1Int=on  enableCEVT2Int=on  enableCEVT3Int=off  enableCEVT4Int=off  enableCTROVFInt=on  enablePRDInt=off  enableCMPInt=off
  eCAP_Out : Outport
  wires:
  eCAP/1 -> eCAP_Out/1

== system mcb_pmsm_foc_hall_f28379d/Hall Sensor A/eCAP/Simulation ==
  Ground : Ground
  Ground1 : Ground
  Mux : Mux  Inputs=2
  eCAP_Out : Outport
  wires:
  Ground1/1 -> Mux/2
  Mux/1 -> eCAP_Out/1
  Ground/1 -> Mux/1

== system mcb_pmsm_foc_hall_f28379d/Hall Sensor B/Capture Event Selection/Output 0 ==
  Action Port : ActionPort  ActionPortLabel=else
  Constant : Constant  Value=0  OutDataTypeStr=boolean
  Out1 : Outport
  wires:
  Constant/1 -> Out1/1

== system mcb_pmsm_foc_hall_f28379d/Hall Sensor B/Capture Event Selection/Output 1 ==
  Action Port : ActionPort  ActionPortLabel=if((u1 == 3 | u1 == 6))
  Constant : Constant  OutDataTypeStr=boolean
  Out1 : Outport
  wires:
  Constant/1 -> Out1/1

== system mcb_pmsm_foc_hall_f28379d/Hall Sensor B/HallValidity/CodeGen ==
  Data Type Conversion : DataTypeConversion  OutDataTypeStr=uint32  ConvertRealWorld=Stored Integer (SI)  SaturateOnIntegerOverflow=off  RndMeth=Floor
  Read Halls : Subsystem  mask(Hall sensor reader){sample_time=-1}
      mask prompts: sample_time "Sample time:"
      mask help:
      | This block outputs the state of the 3 hall sensors placed on GPIO54, 55 and 57 of LaunchXL-F28379D board.
      |
      | 0 --> GPIO57 = 0, GPIO55 = 0, GPIO54 = 0
      | 1 --> GPIO57 = 0, GPIO55 = 0, GPIO54 = 1
      | 2 --> GPIO57 = 0, GPIO55 = 1, GPIO54 = 0
      | 3 --> GPIO57 = 0, GPIO55 = 1, GPIO54 = 1
      | 4 --> GPIO57 = 1, GPIO55 = 0, GPIO54 = 0
      | 5 --> GPIO57 = 1, GPIO55 = 0, GPIO54 = 1
      | 6 --> GPIO57 = 1, GPIO55 = 1, GPIO54 = 0
      | 7 --> GPIO57 = 1, GPIO55 = 1, GPIO54 = 1
  Out1 : Outport
  wires:
  Read Halls/1(Halls) -> Data Type Conversion/1
  Data Type Conversion/1 -> Out1/1

== system mcb_pmsm_foc_hall_f28379d/Hall Sensor B/HallValidity/Sim ==
  Data Type Conversion : DataTypeConversion  OutDataTypeStr=uint32  ConvertRealWorld=Stored Integer (SI)  SaturateOnIntegerOverflow=off  RndMeth=Floor
  Ground : Ground
  Out1 : Outport
  wires:
  Data Type Conversion/1 -> Out1/1
  Ground/1 -> Data Type Conversion/1

== system mcb_pmsm_foc_hall_f28379d/Hall Sensor B/eCAP/Code generation ==
  eCAP : c280xlib/eCAP  operatingMode=eCAP  selectCAPx=eCAP2  offsetValue=0  counterSynIn=off  enableCounter=off  syncOutput=Disabled  sampleTime=-1  eventPrescaler=0  selectMode=Continuous  enableOneShot=off  stopValue=Capture Event 2  resetEv1Ts=on  ev1Polarity=Rising Edge  resetEv2Ts=on  ev2Polarity=Falling Edge  resetEv3Ts=off  ev3Polarity=Rising Edge  resetEv4Ts=off  ev4Polarity=Rising Edge  tSCntrDataType=uint32  capEvFlag=off  capFlagDataType=uint16  overFlowFlag=off  overFlowFlagDataType=uint16  periodUnit=Seconds  periodSource=Specify via dialog  waveformPeriod=0.001  dutyUnit=Percentages  dutySource=Specify via dialog  dutyCycle=50  outputPolarity=Active High  enableCEVT1Int=on  enableCEVT2Int=on  enableCEVT3Int=off  enableCEVT4Int=off  enableCTROVFInt=on  enablePRDInt=off  enableCMPInt=off
  eCAP_Out : Outport
  wires:
  eCAP/1 -> eCAP_Out/1

== system mcb_pmsm_foc_hall_f28379d/Hall Sensor B/eCAP/Simulation ==
  Ground : Ground
  Ground1 : Ground
  Mux : Mux  Inputs=2
  eCAP_Out : Outport
  wires:
  Ground1/1 -> Mux/2
  Mux/1 -> eCAP_Out/1
  Ground/1 -> Mux/1

== system mcb_pmsm_foc_hall_f28379d/Hall Sensor C/Capture Event Selection/Output 0 ==
  Action Port : ActionPort  ActionPortLabel=else
  Constant : Constant  Value=0  OutDataTypeStr=boolean
  Out1 : Outport
  wires:
  Constant/1 -> Out1/1

== system mcb_pmsm_foc_hall_f28379d/Hall Sensor C/Capture Event Selection/Output 1 ==
  Action Port : ActionPort  ActionPortLabel=if((u1 == 5 | u1 == 6))
  Constant : Constant  OutDataTypeStr=boolean
  Out1 : Outport
  wires:
  Constant/1 -> Out1/1

== system mcb_pmsm_foc_hall_f28379d/Hall Sensor C/HallValidity/CodeGen ==
  Data Type Conversion : DataTypeConversion  OutDataTypeStr=uint32  ConvertRealWorld=Stored Integer (SI)  SaturateOnIntegerOverflow=off  RndMeth=Floor
  Read Halls : Subsystem  mask(Hall sensor reader){sample_time=-1}
      mask prompts: sample_time "Sample time:"
      mask help:
      | This block outputs the state of the 3 hall sensors placed on GPIO54, 55 and 57 of LaunchXL-F28379D board.
      |
      | 0 --> GPIO57 = 0, GPIO55 = 0, GPIO54 = 0
      | 1 --> GPIO57 = 0, GPIO55 = 0, GPIO54 = 1
      | 2 --> GPIO57 = 0, GPIO55 = 1, GPIO54 = 0
      | 3 --> GPIO57 = 0, GPIO55 = 1, GPIO54 = 1
      | 4 --> GPIO57 = 1, GPIO55 = 0, GPIO54 = 0
      | 5 --> GPIO57 = 1, GPIO55 = 0, GPIO54 = 1
      | 6 --> GPIO57 = 1, GPIO55 = 1, GPIO54 = 0
      | 7 --> GPIO57 = 1, GPIO55 = 1, GPIO54 = 1
  Out1 : Outport
  wires:
  Data Type Conversion/1 -> Out1/1
  Read Halls/1(Halls) -> Data Type Conversion/1

== system mcb_pmsm_foc_hall_f28379d/Hall Sensor C/HallValidity/Sim ==
  Data Type Conversion : DataTypeConversion  OutDataTypeStr=uint32  ConvertRealWorld=Stored Integer (SI)  SaturateOnIntegerOverflow=off  RndMeth=Floor
  Ground : Ground
  Out1 : Outport
  wires:
  Data Type Conversion/1 -> Out1/1
  Ground/1 -> Data Type Conversion/1

== system mcb_pmsm_foc_hall_f28379d/Hall Sensor C/eCAP/Code generation ==
  eCAP : c280xlib/eCAP  operatingMode=eCAP  selectCAPx=eCAP3  offsetValue=0  counterSynIn=off  enableCounter=off  syncOutput=Disabled  sampleTime=-1  eventPrescaler=0  selectMode=Continuous  enableOneShot=off  stopValue=Capture Event 2  resetEv1Ts=on  ev1Polarity=Rising Edge  resetEv2Ts=on  ev2Polarity=Falling Edge  resetEv3Ts=off  ev3Polarity=Rising Edge  resetEv4Ts=off  ev4Polarity=Rising Edge  tSCntrDataType=uint32  capEvFlag=off  capFlagDataType=uint16  overFlowFlag=off  overFlowFlagDataType=uint16  periodUnit=Seconds  periodSource=Specify via dialog  waveformPeriod=0.001  dutyUnit=Percentages  dutySource=Specify via dialog  dutyCycle=50  outputPolarity=Active High  enableCEVT1Int=on  enableCEVT2Int=on  enableCEVT3Int=off  enableCEVT4Int=off  enableCTROVFInt=on  enablePRDInt=off  enableCMPInt=off
  eCAP_Out : Outport
  wires:
  eCAP/1 -> eCAP_Out/1

== system mcb_pmsm_foc_hall_f28379d/Hall Sensor C/eCAP/Simulation ==
  Ground : Ground
  Ground1 : Ground
  Mux : Mux  Inputs=2
  eCAP_Out : Outport
  wires:
  Ground1/1 -> Mux/2
  Mux/1 -> eCAP_Out/1
  Ground/1 -> Mux/1

== system mcb_pmsm_foc_hall_f28379d/Hardware Init/Variant Subsystem/Code Generation ==
  In1 : Inport
  ADC Calib Enable : Constant  Value=inverter.ADCOffsetCalibEnable  OutDataTypeStr=Inherit: Inherit via back propagation
  "Calculate ADC Offset " : Subsystem  Priority=1001  TreatAsAtomicUnit=on
  DRV Enable : Subsystem  Priority=1
  Default ADC Offset : Subsystem  Priority=1001  TreatAsAtomicUnit=on
  NOT : Logic  Operator=NOT  IconShape=distinctive  AllPortsSameDT=off  OutDataTypeStr=boolean
  wires:
  In1/1 -> DRV Enable/1(In)
  NOT/1 -> Default ADC Offset/Enable
  ADC Calib Enable/1 -> NOT/1, "Calculate ADC Offset "/Enable

== system mcb_pmsm_foc_hall_f28379d/Hardware Init/Variant Subsystem/Simulation ==
  In1 : Inport
  Terminator : Terminator
  wires:
  In1/1 -> Terminator/1

== system mcb_pmsm_foc_hall_f28379d/Heartbeat LED/Heartbeat LED/Code generation ==
  In1 : Inport
  Digital Output2 : c2837xDlib/Digital Output  GPIO_Number=GPIO32~GPIO39  GPIO_Bit0=off  GPIO_BIT0_Toggle=on  GPIO_Bit1=off  GPIO_BIT1_Toggle=off  GPIO_Bit2=on  GPIO_BIT2_Toggle=on  GPIO_Bit3=off  GPIO_BIT3_Toggle=off  GPIO_Bit4=off  GPIO_BIT4_Toggle=off  GPIO_Bit5=off  GPIO_BIT5_Toggle=off  GPIO_Bit6=off  GPIO_BIT6_Toggle=off  GPIO_Bit7=off  GPIO_BIT7_Toggle=on
  wires:
  In1/1 -> Digital Output2/1

== system mcb_pmsm_foc_hall_f28379d/Heartbeat LED/Heartbeat LED/Simulation ==
  In1 : Inport
  Simulation_Terminator : Terminator
  wires:
  In1/1 -> Simulation_Terminator/1

== system mcb_pmsm_foc_hall_f28379d/Inverter and Motor - Plant Model/Simulation/Inverter ==
  Duty_abc : Inport
  Average-Value Inverter : mcbplantlib/Average-Value Inverter
  Constant2 : Constant  Value=inverter.V_dc  OutDataTypeStr=single  SampleTime=-1
  Data Type Conversion1 : DataTypeConversion  OutDataTypeStr=single  RndMeth=Simplest  SaturateOnIntegerOverflow=off
  Rate Transition3 : RateTransition  Integrity=off  OutPortSampleTime=Ts_inverter
  Vabc : Outport  VectorParamsAs1DForOutWhenUnconnected=off
  wires:
  Duty_abc/1 -> Data Type Conversion1/1
  Data Type Conversion1/1 -> Rate Transition3/1
  Rate Transition3/1 -> Average-Value Inverter/1
  Constant2/1 -> Average-Value Inverter/2
  Average-Value Inverter/1 -> Vabc/1

== system mcb_pmsm_foc_hall_f28379d/Inverter and Motor - Plant Model/Simulation/Load_Profile (Torque) ==
  Data Type Conversion : DataTypeConversion  OutDataTypeStr=single  SaturateOnIntegerOverflow=off  RndMeth=Floor
  IIR Filter : mcbcontrolslib/IIR Filter  VariantControl=Low Pass Filter  VariantSelect=Low-pass  Filter_constant=0.01  advancedSettings=off  Ts=50e-6  cutOff_freq=32.1525
  T_load : Step  Time=5  Before=0.05*pmsm.T_rated  After=0.5*pmsm.T_rated  SampleTime=Ts_simulink
  Load_Trq : Outport  VectorParamsAs1DForOutWhenUnconnected=off
  wires:
  T_load/1 -> Data Type Conversion/1
  Data Type Conversion/1 -> IIR Filter/1
  IIR Filter/1 -> Load_Trq/1

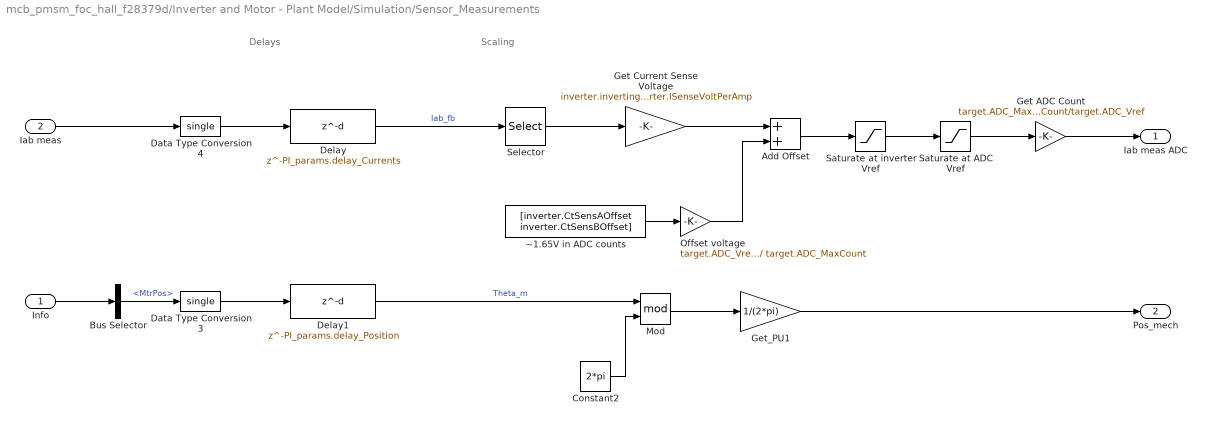
== system mcb_pmsm_foc_hall_f28379d/Inverter and Motor - Plant Model/Simulation/Sensor_Measurements ==
  note: Scaling
  note: Delays
  Info : Inport
  Iab meas : Inport  Port=2
  Add Offset : Sum  RndMeth=Simplest
  Bus Selector : BusSelector  OutputSignals=MtrPos
  Constant2 : Constant  Value=2*pi  OutDataTypeStr=single  SampleTime=-1
  Data Type Conversion3 : DataTypeConversion  OutDataTypeStr=single  RndMeth=Simplest  SaturateOnIntegerOverflow=off
  Data Type Conversion4 : DataTypeConversion  OutDataTypeStr=single  RndMeth=Simplest  SaturateOnIntegerOverflow=off
  Delay : Delay  DelayLength=PI_params.delay_Currents
  Delay1 : Delay  DelayLength=PI_params.delay_Position
  Get ADC Count : Gain  Gain=target.ADC_MaxCount/target.ADC_Vref  OutMin=0  OutMax=target.ADC_MaxCount  OutDataTypeStr=uint16  RndMeth=Simplest
  Get Current Sense Voltage : Gain  Gain=inverter.invertingAmp * inverter.ISenseVoltPerAmp  RndMeth=Simplest  OutDataTypeStr=Inherit: Same as input
  Get_PU1 : Gain  Gain=1/(2*pi)  OutDataTypeStr=dataType  RndMeth=Simplest
  Mod : Math  Operator=mod
  Offset voltage : Gain  Gain=target.ADC_Vref / target.ADC_MaxCount  RndMeth=Simplest
  Saturate at ADC Vref : Saturate  UpperLimit=target.ADC_Vref  LowerLimit=0
  Saturate at inverter Vref : Saturate  UpperLimit=inverter.ISenseVref  LowerLimit=0
  Selector : Selector  InputPortWidth=3  IndexOptions=Index vector (dialog)  Indices=[1 2]  OutputSizes=1
  ~1.65V in ADC counts : Constant  Value=[inverter.CtSensAOffset inverter.CtSensBOffset]  OutDataTypeStr=uint16  SampleTime=-1
  Iab meas ADC : Outport  VectorParamsAs1DForOutWhenUnconnected=off
  Pos_mech : Outport  Port=2
  wires:
  Delay/1 -> Selector/1  "Iab_fb"
  Data Type Conversion4/1 -> Delay/1
  Iab meas/1 -> Data Type Conversion4/1
  Info/1 -> Bus Selector/1
  Data Type Conversion3/1 -> Delay1/1
  Get_PU1/1 -> Pos_mech/1
  Bus Selector/1 -> Data Type Conversion3/1  "<MtrPos>"
  Constant2/1 -> Mod/2
  Mod/1 -> Get_PU1/1
  Delay1/1 -> Mod/1  "Theta_m"
  Selector/1 -> Get Current Sense Voltage/1
  Saturate at inverter Vref/1 -> Saturate at ADC Vref/1
  Add Offset/1 -> Saturate at inverter Vref/1
  Get ADC Count/1 -> Iab meas ADC/1
  Offset voltage/1 -> Add Offset/2
  Saturate at ADC Vref/1 -> Get ADC Count/1
  ~1.65V in ADC counts/1 -> Offset voltage/1
  Get Current Sense Voltage/1 -> Add Offset/1

== system mcb_pmsm_foc_hall_f28379d/Serial Receive/Data_Conditioning_Rx/Data_Type_Fixed_Point ==
  In1 : Inport
  Data Type Conversion1 : DataTypeConversion  OutDataTypeStr=dataType  RndMeth=Simplest  SaturateOnIntegerOverflow=off
  Data Type Conversion2 : DataTypeConversion  OutDataTypeStr=fixdt(1,32,28)  ConvertRealWorld=Stored Integer (SI)  RndMeth=Simplest  SaturateOnIntegerOverflow=off
  Data Type Conversion3 : DataTypeConversion  OutDataTypeStr=uint16  RndMeth=Simplest  SaturateOnIntegerOverflow=off
  Demux : Demux  Outputs=2
  Desired Speed : Outport
  Out2 : Outport  Port=2
  wires:
  In1/1 -> Demux/1
  Data Type Conversion1/1 -> Desired Speed/1
  Data Type Conversion2/1 -> Data Type Conversion1/1
  Demux/1 -> Data Type Conversion2/1
  Demux/2 -> Data Type Conversion3/1
  Data Type Conversion3/1 -> Out2/1
